simulink model "final"  (R2024a)
settings: Solver=FixedStepAuto  StartTime=0.0  StopTime=.35  FixedStep=1/f_simu  RelTol=1e-3
InitFcn:
  | % DC motor parameters
  | UaN = 140;          % rated voltage                     V
  | IaN = 25;           % rated current                     A
  | PN = 3336;          % power                             W
  | La = 1.7e-3;        % amature inductance                H
  | Ra = 0.26;          % amature resistance                Ohm
  | TN = 0.26;          % rated load                        N
  | nN = 3000;          % rated angular velocity            rpm
  | J = 0.00252;        % moment of inertia                 kg.m^2
  | B = 0;              % coefficient of viscous friction   kg.m^2/sec
  | 
  | % Unknown parameters calculating
  | KE = (UaN - Ra*IaN)*9.55/nN ;
  | KT = KE;
  | 
  | % PI current controller
  | fsw = 5e4;
  | w_cc = fsw/20;
  | Kpc = La*w_cc;
  | Kic = Ra*w_cc;
  | Kac = 1/Kpc;
  | 
  | % PI speed controller
  | w_cs = w_cc/5;
  | Kps = J*w_cs/KT;
  | Kis = J*w_cs^2/(5*KT);
  | Kas = 1/Kps;
  | 
  | % Simulink sampling freq
  | f_simu = 1e6;
libraries: spsMosfetLib x12, spsDCVoltageSourceLib x3, spsVoltageMeasurementLib x3, simulink x3, spsDCMachineLib x2, spspowerguiLib x1
settings Model: Creator=luand  LastModifiedBy=luand
settings RTWCC: GPUComputeCapability=3.5

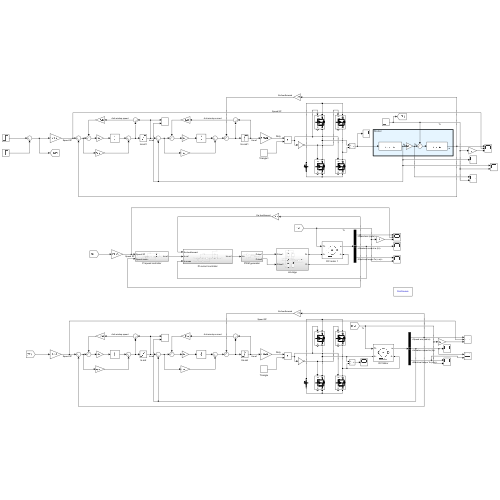
[thumbnail: Simulink's stored preview of the top-level diagram]
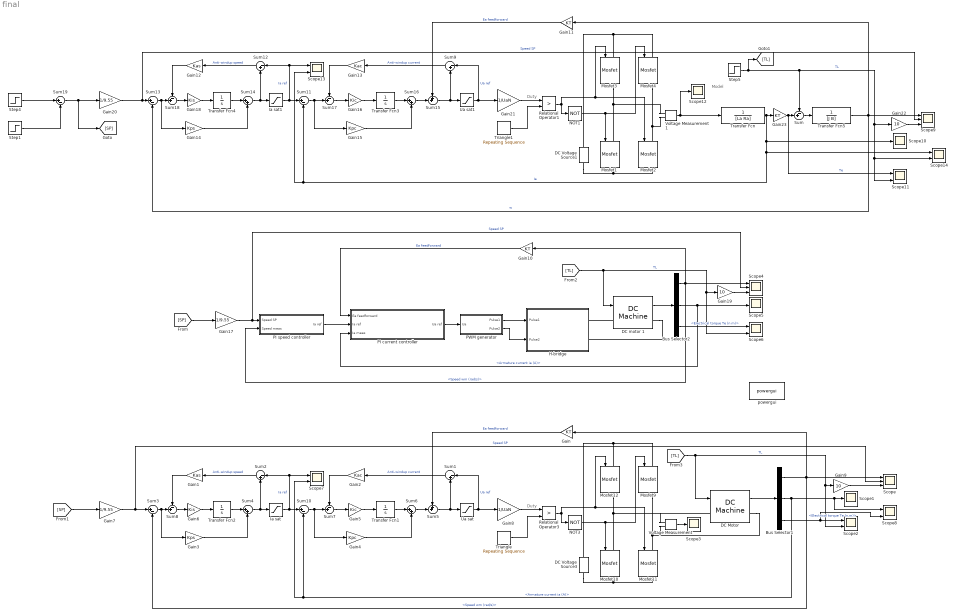
== system final ==
  note: Duty
  note: Duty
  note: Model
  Bus Selector1 : BusSelector  OutputSignals=Speed wm (rad/s),Armature current ia (A),Electrical torque Te (n m)
  Bus Selector2 : BusSelector  OutputSignals=Speed wm (rad/s),Armature current ia (A),Electrical torque Te (n m)
  DC Motor : spsDCMachineLib/DC Machine  PresetModel=No  MechanicalLoad=Torque TL  FieldType=Permanent magnet  ShowDetailedParameters=on  MeasurementBus=off  RLa=[ Ra La ]  RLf="[ 240  120]"  Laf=1.8  MachineConstant=Torque constant (N.m/A)  Ke=1.8  Kt=KT  J=J  Bm=0  Tf=0  w0=0  Ifinit=1  TsPowergui=0  TsBlock=-1
  DC Voltage Source1 : spsDCVoltageSourceLib/DC Voltage Source  Amplitude=UaN  Measurements=None
  DC Voltage Source3 : spsDCVoltageSourceLib/DC Voltage Source  Amplitude=UaN  Measurements=None
  DC motor 1 : spsDCMachineLib/DC Machine  PresetModel=No  MechanicalLoad=Torque TL  FieldType=Permanent magnet  ShowDetailedParameters=on  MeasurementBus=off  RLa=[ Ra La ]  RLf="[ 240  120]"  Laf=1.8  MachineConstant=Torque constant (N.m/A)  Ke=1.8  Kt=KT  J=J  Bm=0  Tf=0  w0=0  Ifinit=1  TsPowergui=0  TsBlock=-1
  Gain{,10..11,23} (4 alike) : Gain  Gain=KT
  Gain1 : Gain  Gain=Kas
  Gain12 : Gain  Gain=Kas
  Gain13 : Gain  Gain=Kac
  Gain14 : Gain  Gain=Kps
  Gain15 : Gain  Gain=Kpc
  Gain16 : Gain  Gain=Kic
  Gain17 : Gain  Gain=1/9.55
  Gain18 : Gain  Gain=Kis
  Gain19 : Gain  Gain=10
  Gain2 : Gain  Gain=Kac
  Gain20 : Gain  Gain=1/9.55
  Gain21 : Gain  Gain=1/UaN
  Gain22 : Gain  Gain=10
  Gain3 : Gain  Gain=Kps
  Gain4 : Gain  Gain=Kpc
  Gain5 : Gain  Gain=Kic
  Gain6 : Gain  Gain=Kis
  Gain7 : Gain  Gain=1/9.55
  Gain8 : Gain  Gain=1/UaN
  Gain9 : Gain  Gain=10
  H-bridge : Subsystem
  Ia sat : Saturate  UpperLimit=IaN*8  LowerLimit=-IaN*8
  Ia sat1 : Saturate  UpperLimit=IaN*8  LowerLimit=-IaN*8
  Mosfet{1..4,9..12} (8 alike) : spsMosfetLib/Mosfet  Ron=1e-3  Lon=0  Rd=0.01  Vfd=0  IC=0  Rs=1e5  Cs=inf  Measurements=on
  NOT1 : Logic  Operator=NOT  IconShape=distinctive  AllPortsSameDT=off  OutDataTypeStr=boolean
  NOT3 : Logic  Operator=NOT  IconShape=distinctive  AllPortsSameDT=off  OutDataTypeStr=boolean
  PI current controller : Subsystem
  PI speed controller : Subsystem
  PWM generator : Subsystem
  Relational Operator1 : RelationalOperator  Operator=>  OutDataTypeStr=boolean  RndMeth=Simplest  InputSameDT=off
  Relational Operator3 : RelationalOperator  Operator=>  OutDataTypeStr=boolean  RndMeth=Simplest  InputSameDT=off
  Scope : Scope  NumInputPorts=3
  Scope{1,3,5,10,12} (5 alike) : Scope
  Scope{2,6..8,11,13..14} (7 alike) : Scope  NumInputPorts=2
  Scope4 : Scope  NumInputPorts=3
  Scope9 : Scope  NumInputPorts=3
  Step1 : Step  Time=.25  After=1000  SampleTime=0
  Step4 : Step  Time=.1  Before=-2500  After=3000  SampleTime=0
  Step5 : Step  Time=.2  After=30  SampleTime=0
  Sum{,7..8,17..18} (5 alike) : Sum  Inputs=-+|
  Sum{1..2,9,12} (4 alike) : Sum  Inputs=|-+
  Sum{3,10..11,13,19} (5 alike) : Sum  Inputs=|+-
  Sum{4,6,14,16} (4 alike) : Sum  Inputs=|++
  Sum15 : Sum  Inputs=++|
  Sum5 : Sum  Inputs=++|
  Transfer Fcn : TransferFcn  Denominator=[La Ra]
  Transfer Fcn{1..4} (4 alike) : TransferFcn  Denominator=[1 0]
  Transfer Fcn5 : TransferFcn  Denominator=[J B]
  Triangle : simulink/Sources/Repeating Sequence  rep_seq_t=[0 1e-5 1/fsw]  rep_seq_y=[-1 1 -1]
  Triangle1 : simulink/Sources/Repeating Sequence  rep_seq_t=[0 1/(fsw*2) 1/fsw]  rep_seq_y=[-1 1 -1]
  Ua sat : Saturate  UpperLimit=UaN  LowerLimit=-UaN
  Ua sat1 : Saturate  UpperLimit=UaN  LowerLimit=-UaN
  Voltage Measurement : spsVoltageMeasurementLib/Voltage Measurement  PhasorSimulation=off  OutputType=Complex  PSBequivalent=0
  Voltage Measurement1 : spsVoltageMeasurementLib/Voltage Measurement  PhasorSimulation=off  OutputType=Complex  PSBequivalent=0
  powergui : spspowerguiLib/powergui  Priority=1  SimulationMode=Continuous  SampleTime=50e-6  frequency=60  Iterations=50  frequencyindice=0  Pbase=100e6  ErrMax=1e-4  UnitsV=kV  UnitsW=MW  buscounter=0  FunctionMessages=off  echomessages=off  EnableUseOfTLC=off  CurrentSourceSwitches=off  DisableSnubberDevices=off  DisableRonSwitches=off  DisableVfSwitches=off  DisplayEquations=off  AutomaticDiscreteSolvers=off  SolverType=Tustin/Backward Euler (TBE)  Interpol=off  ExternalGateDelay=off  methode=off  Ts=100  x0status=blocks  SPID=on  SwTol=0  HookPort=off  NonlinearTolerance=1e-4  nMaxIteration=100  ContinueOnMaxIteration=off  RestoreLinks=warning  ResistiveCurrentMeasurement=off  Frange=[0:2:500]  Ylog=off  Xlog=on  ShowGrid=off  save=off  variable=ZData  structure=0  ZoomFFT=off  StartTime=0.0  cycles=1  DisplayStyle=1  fundamental=60  FreqAxis=off  MaxFrequency=1000  frequencyindicesteady=1  RmsSteady=1  display=off
  wires:
  DC Motor/1 -> Bus Selector1/1
  Bus Selector1/1 -> Scope/1, Sum3/2, Gain/1  "<Speed wm (rad/s)>"
  Sum1/1 -> Gain2/1  "Anti-windup current"
  Sum5/1 -> Ua sat/1, Sum1/2
  Gain5/1 -> Transfer Fcn1/1
  Sum7/1 -> Gain5/1
  Sum6/1 -> Sum5/2
  Transfer Fcn1/1 -> Sum6/1
  Gain4/1 -> Sum6/2
  Gain2/1 -> Sum7/1
  Ua sat/1 -> Gain8/1, Sum1/1  "Ua ref"
  Gain/1 -> Sum5/1  "Ea feedforward"
  Bus Selector1/2 -> Scope8/1, Scope1/1, Sum10/2, Scope7/2  "<Armature current ia (A)>"
  Sum10/1 -> Sum7/2, Gain4/1
  Sum3/1 -> Gain3/1, Sum8/2
  Sum4/1 -> Ia sat/1, Sum2/2
  Gain3/1 -> Sum4/2
  Transfer Fcn2/1 -> Sum4/1
  Sum8/1 -> Gain6/1
  Gain6/1 -> Transfer Fcn2/1
  Sum2/1 -> Gain1/1  "Anti-windup speed"
  [SP] -> Gain7/1
  Relational Operator3/1 -> NOT3/1, Mosfet11/1, Mosfet12/1
  Triangle/1 -> Relational Operator3/2
  NOT3/1 -> Mosfet10/1, Mosfet9/1
  Gain8/1 -> Relational Operator3/1
  [TL] -> DC Motor/1, Gain9/1, Scope2/2  "TL"
  Bus Selector1/3 -> Scope8/2, Scope2/1  "<Electrical torque Te (n m)>"
  Gain9/1 -> Scope/3
  Ia sat/1 -> Sum10/1, Scope7/1, Sum2/1  "Ia ref"
  Voltage Measurement/1 -> Scope3/1
  Gain1/1 -> Sum8/1
  Gain7/1 -> Scope/2, Sum3/1  "Speed SP"
  Gain17/1 -> Scope4/2, PI speed controller/1(Speed SP)  "Speed SP"
  Gain19/1 -> Scope4/3
  Bus Selector2/3 -> Scope6/1  "<Electrical torque Te (n m)>"
  [TL] -> Scope6/2, Gain19/1, DC motor 1/1  "TL"
  [SP] -> Gain17/1
  Bus Selector2/2 -> Scope5/1, PI current controller/3(Ia meas)  "<Armature current ia (A)>"
  Bus Selector2/1 -> Gain10/1, PI speed controller/2(Speed meas), Scope4/1  "<Speed wm (rad/s)>"
  DC motor 1/1 -> Bus Selector2/1
  Gain10/1 -> PI current controller/1(Ea feedforward)  "Ea feedforward"
  PI speed controller/1(Ia ref) -> PI current controller/2(Ia ref)
  PI current controller/1(Ua ref) -> PWM generator/1(Ua)
  PWM generator/1(Pulse1) -> H-bridge/1(Pulse1)
  PWM generator/2(Pulse2) -> H-bridge/2(Pulse2)
  Gain20/1 -> Sum13/1, Scope9/2  "Speed SP"
  Gain12/1 -> Sum18/1
  Voltage Measurement1/1 -> Transfer Fcn/1, Scope12/1
  Ia sat1/1 -> Sum12/1, Scope13/1, Sum11/1  "Ia ref"
  Gain22/1 -> Scope9/3
  Step5/1 -> [TL], Scope11/2, Scope14/2, Gain22/1, Sum/1  "TL"
  Gain21/1 -> Relational Operator1/1
  NOT1/1 -> Mosfet4/1, Mosfet1/1
  Triangle1/1 -> Relational Operator1/2
  Relational Operator1/1 -> Mosfet3/1, Mosfet2/1, NOT1/1
  Sum12/1 -> Gain12/1  "Anti-windup speed"
  Gain18/1 -> Transfer Fcn4/1
  Sum18/1 -> Gain18/1
  Transfer Fcn4/1 -> Sum14/1
  Gain14/1 -> Sum14/2
  Sum14/1 -> Sum12/2, Ia sat1/1
  Sum13/1 -> Sum18/2, Gain14/1
  Sum11/1 -> Gain15/1, Sum17/2
  Gain11/1 -> Sum15/1  "Ea feedforward"
  Ua sat1/1 -> Sum9/1, Gain21/1  "Ua ref"
  Gain13/1 -> Sum17/1
  Gain15/1 -> Sum16/2
  Transfer Fcn3/1 -> Sum16/1
  Sum16/1 -> Sum15/2
  Sum17/1 -> Gain16/1
  Gain16/1 -> Transfer Fcn3/1
  Sum15/1 -> Sum9/2, Ua sat1/1
  Sum9/1 -> Gain13/1  "Anti-windup current"
  Sum/1 -> Transfer Fcn5/1
  Transfer Fcn/1 -> Scope14/1, Scope13/2, Sum11/2, Scope10/1, Gain23/1  "Ia"
  Gain23/1 -> Scope11/1, Sum/2  "Te"
  Transfer Fcn5/1 -> Scope9/1, Sum13/2, Gain11/1  "w"
  Step4/1 -> Sum19/1
  Sum19/1 -> [SP], Gain20/1
  Step1/1 -> Sum19/2
  connections:
  Mosfet9/RConn1 -- Voltage Measurement/LConn2 -- DC Motor/RConn1 -- Mosfet11/LConn1
  Mosfet10/RConn1 -- DC Voltage Source3/LConn1 -- Mosfet11/RConn1
  Mosfet12/LConn1 -- DC Voltage Source3/RConn1 -- Mosfet9/LConn1
  Mosfet12/RConn1 -- Voltage Measurement/LConn1 -- DC Motor/LConn1 -- Mosfet10/LConn1
  DC motor 1/LConn1 -- H-bridge/RConn1
  DC motor 1/RConn1 -- H-bridge/RConn2
  Mosfet4/RConn1 -- Voltage Measurement1/LConn2 -- Mosfet2/LConn1
  Mosfet1/RConn1 -- DC Voltage Source1/LConn1 -- Mosfet2/RConn1
  Mosfet3/LConn1 -- DC Voltage Source1/RConn1 -- Mosfet4/LConn1
  Mosfet3/RConn1 -- Voltage Measurement1/LConn1 -- Mosfet1/LConn1

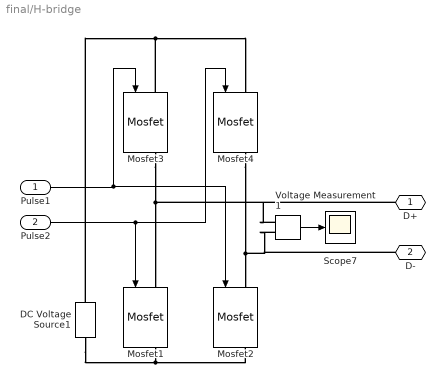
== system final/H-bridge ==
  Pulse1 : Inport
  Pulse2 : Inport  Port=2
  DC Voltage Source1 : spsDCVoltageSourceLib/DC Voltage Source  Amplitude=UaN  Measurements=None
  Mosfet{1..4} (4 alike) : spsMosfetLib/Mosfet  Ron=1e-3  Lon=0  Rd=0.01  Vfd=0  IC=0  Rs=1e5  Cs=inf  Measurements=on
  Scope7 : Scope
  Voltage Measurement1 : spsVoltageMeasurementLib/Voltage Measurement  PhasorSimulation=off  OutputType=Complex  PSBequivalent=0
  D+ : PMIOPort  Side=Right
  D- : PMIOPort  Port=2  Side=Right
  wires:
  Pulse2/1 -> Mosfet4/1, Mosfet1/1
  Voltage Measurement1/1 -> Scope7/1
  Pulse1/1 -> Mosfet3/1, Mosfet2/1
  connections:
  Mosfet1/RConn1 -- Mosfet2/RConn1 -- DC Voltage Source1/LConn1
  Mosfet4/RConn1 -- D-/RConn1 -- Voltage Measurement1/LConn2 -- Mosfet2/LConn1
  Mosfet3/LConn1 -- Mosfet4/LConn1 -- DC Voltage Source1/RConn1
  Mosfet3/RConn1 -- Mosfet1/LConn1 -- D+/RConn1 -- Voltage Measurement1/LConn1

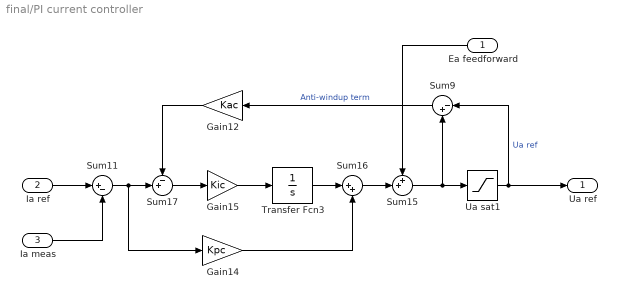
== system final/PI current controller ==
  Ea feedforward : Inport
  Ia ref : Inport  Port=2
  Ia meas : Inport  Port=3
  Gain12 : Gain  Gain=Kac
  Gain14 : Gain  Gain=Kpc
  Gain15 : Gain  Gain=Kic
  Sum11 : Sum  Inputs=|+-
  Sum15 : Sum  Inputs=++|
  Sum16 : Sum  Inputs=|++
  Sum17 : Sum  Inputs=-+|
  Sum9 : Sum  Inputs=|-+
  Transfer Fcn3 : TransferFcn  Denominator=[1 0]
  Ua sat1 : Saturate  UpperLimit=UaN  LowerLimit=-UaN
  Ua ref : Outport
  wires:
  Gain12/1 -> Sum17/1
  Sum11/1 -> Gain14/1, Sum17/2
  Sum16/1 -> Sum15/2
  Ua sat1/1 -> Ua ref/1, Sum9/1  "Ua ref"
  Sum15/1 -> Sum9/2, Ua sat1/1
  Gain15/1 -> Transfer Fcn3/1
  Sum17/1 -> Gain15/1
  Sum9/1 -> Gain12/1  "Anti-windup term"
  Gain14/1 -> Sum16/2
  Transfer Fcn3/1 -> Sum16/1
  Ea feedforward/1 -> Sum15/1
  Ia meas/1 -> Sum11/2
  Ia ref/1 -> Sum11/1

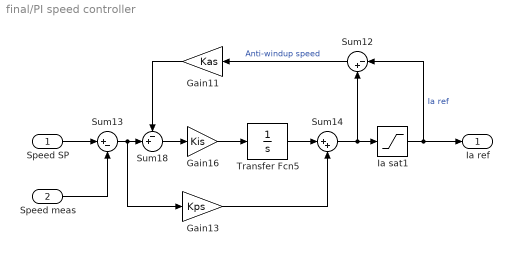
== system final/PI speed controller ==
  Speed SP : Inport
  Speed meas : Inport  Port=2
  Gain11 : Gain  Gain=Kas
  Gain13 : Gain  Gain=Kps
  Gain16 : Gain  Gain=Kis
  Ia sat1 : Saturate  UpperLimit=IaN*7  LowerLimit=-IaN*7
  Sum12 : Sum  Inputs=|-+
  Sum13 : Sum  Inputs=|+-
  Sum14 : Sum  Inputs=|++
  Sum18 : Sum  Inputs=-+|
  Transfer Fcn5 : TransferFcn  Denominator=[1 0]
  Ia ref : Outport
  wires:
  Gain11/1 -> Sum18/1
  Transfer Fcn5/1 -> Sum14/1
  Sum13/1 -> Sum18/2, Gain13/1
  Sum14/1 -> Sum12/2, Ia sat1/1
  Ia sat1/1 -> Ia ref/1, Sum12/1  "Ia ref"
  Gain13/1 -> Sum14/2
  Sum12/1 -> Gain11/1  "Anti-windup speed"
  Gain16/1 -> Transfer Fcn5/1
  Sum18/1 -> Gain16/1
  Speed SP/1 -> Sum13/1
  Speed meas/1 -> Sum13/2

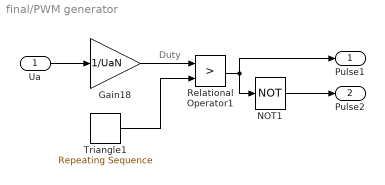
== system final/PWM generator ==
  note: Duty
  Ua : Inport
  Gain18 : Gain  Gain=1/UaN
  NOT1 : Logic  Operator=NOT  IconShape=distinctive  AllPortsSameDT=off  OutDataTypeStr=boolean
  Relational Operator1 : RelationalOperator  Operator=>  OutDataTypeStr=boolean  RndMeth=Simplest  InputSameDT=off
  Triangle1 : simulink/Sources/Repeating Sequence  rep_seq_t=[0 .5e-4 1e-4]  rep_seq_y=[-1 1 -1]
  Pulse1 : Outport
  Pulse2 : Outport  Port=2
  wires:
  Relational Operator1/1 -> Pulse1/1, NOT1/1
  NOT1/1 -> Pulse2/1
  Triangle1/1 -> Relational Operator1/2
  Gain18/1 -> Relational Operator1/1
  Ua/1 -> Gain18/1
